simulink model "OscillatoreVandDerPool"  (R2020b)
settings: Solver=VariableStepAuto  StartTime=0.0  StopTime=100.0  RelTol=1e-3
libraries: simulink x1
settings Model: Creator=loryb  LastModifiedBy=loryb

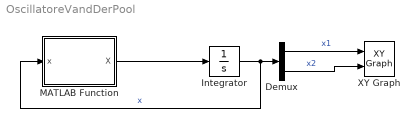
== system OscillatoreVandDerPool ==
  Demux : Demux  Outputs=2
  Integrator : Integrator  InitialCondition=[1;0]
  MATLAB Function : MATLAB Function  TreatAsAtomicUnit=on
  XY Graph : simulink/Sinks/XY Graph  xmin=-1  xmax=1  ymin=-1  ymax=1  st=-1
  wires:
  MATLAB Function/1(X) -> Integrator/1
  Integrator/1 -> MATLAB Function/1(x), Demux/1  "x"
  Demux/1 -> XY Graph/1  "x1"
  Demux/2 -> XY Graph/2  "x2"

== matlab function OscillatoreVandDerPool/MATLAB Function ==
  data: x input; X output
function X = fcn(x)
eps = -0.01;
dx1 = x(2);
dx2 = -x(1)-eps*(-1+x(1)^2)*x(2);
X = [dx1;dx2];
